simulink model "Copy_of_prvish"  (Simulink 8.6)
settings: Solver=ode45  StartTime=0.0  StopTime=200  RelTol=1e-3
libraries: fuzblock x1
settings Model: Creator=iki  LastModifiedBy=Branko
settings DebuggingCC: FcnCallInpInsideContextMsg=EnableAllAsWarning

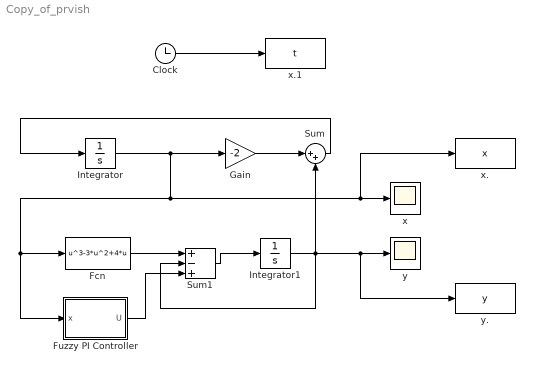
== system Copy_of_prvish ==
  Clock : Clock
  Fcn : Fcn  Expr=u^3-3*u^2+4*u
  Fuzzy PI Controller : Subsystem
  Gain : Gain  Gain=-2
  Integrator : Integrator  InitialCondition=-2
  Integrator1 : Integrator  InitialCondition=8
  Sum : Sum  Inputs=|++
  Sum1 : Sum  Inputs=+-+
  x : Scope
  x. : ToWorkspace  VariableName=x  SampleTime=-1
      settings: Save2DSignal=2-D array (concatenate along first dimension)
  x.1 : ToWorkspace  VariableName=t  SampleTime=-1
      settings: Save2DSignal=2-D array (concatenate along first dimension)
  y : Scope
  y. : ToWorkspace  VariableName=y  SampleTime=-1
      settings: Save2DSignal=2-D array (concatenate along first dimension)
  wires:
  Integrator/1 -> Gain/1, x/1, x./1, Fcn/1, Fuzzy PI Controller/1(x)
  Gain/1 -> Sum/1
  Sum/1 -> Integrator/1
  Integrator1/1 -> Sum/2, Sum1/2, y/1, y./1
  Sum1/1 -> Integrator1/1
  Fcn/1 -> Sum1/1
  Fuzzy PI Controller/1(U) -> Sum1/3
  Clock/1 -> x.1/1

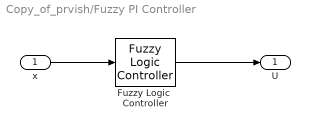
== system Copy_of_prvish/Fuzzy PI Controller ==
  x : Inport
  Fuzzy Logic  Controller : fuzblock/Fuzzy Logic  Controller  fis=fuzzyPI1
  U : Outport
  wires:
  x/1 -> Fuzzy Logic  Controller/1
  Fuzzy Logic  Controller/1 -> U/1
